simulink model "nonlinear_crane_example"  (Simulink 8.6)
settings: Solver=VariableStepAuto  SolverMode=SingleTasking  StartTime=0.0  StopTime=10  RelTol=1e-3
InitFcn:
  | nonlinear_crane_example_initfcn
values from neighbouring files (symbols this model uses):
  A_nz_idx = ( 1:1:nnz( Anz ) )    [nonlinear_crane_example_initfcn.m]
  Anz = [Anz ... (first row only)    [nonlinear_crane_example_initfcn.m]
  g = 9.81    [nonlinear_crane_example_initfcn.m]
  lineq = repmat(ls, N, 1)    [nonlinear_crane_example_initfcn.m]
  N = 5    [nonlinear_crane_example_initfcn.m]
  nu = 2    [nonlinear_crane_example_initfcn.m]
  nx = 6    [nonlinear_crane_example_initfcn.m]
  P_nz_idx = ( 1:1:nnz( Pnz ) )    [nonlinear_crane_example_initfcn.m]
  Pnz = blkdiag( Pnz, Q )    [nonlinear_crane_example_initfcn.m]
  q = zeros( 1, length(Pnz) )    [nonlinear_crane_example_initfcn.m]
  tau_c = 0.13    [nonlinear_crane_example_initfcn.m]
  tau_l = 0.07    [nonlinear_crane_example_initfcn.m]
  traj_0 = traj_0( 1:1:(length(traj_0)-nu), : )    [nonlinear_crane_example_initfcn.m]
  u0 = zeros(nu, 1)    [nonlinear_crane_example_initfcn.m]
  uineq = repmat(us, N, 1)    [nonlinear_crane_example_initfcn.m]
  x0 = zeros(nx, 1)    [nonlinear_crane_example_initfcn.m]
libraries: osqp_library x1, simulink x1
settings Model: Creator=im1716  LastModifiedBy=imcinerney
settings DataIOCC: LimitDataPoints=off  SaveFormat=Dataset  SignalLoggingSaveFormat=Dataset  ReturnWorkspaceOutputs=on
settings OptimizationCC: ExpressionDepthLimit=128
settings DebuggingCC: UnderspecifiedInitializationDetection=Simplified  MergeDetectMultiDrivingBlocksExec=error  SolverPrmCheckMsg=none  FcnCallInpInsideContextMsg=EnableAllAsError  AllowSymbolicDim=on  StateNameClashWarn=none  SFUnexpectedBacktrackingDiag=error  SFNoUnconditionalDefaultTransitionDiag=error
settings HardwareCC: ProdBitPerPointer=64  ProdLargestAtomicFloat=Float  ProdIntDivRoundTo=Zero  ProdEndianess=LittleEndian  ProdWordSize=64  ProdHWDeviceType=Intel->x86-64 (Windows64)
settings ModelReferenceCC: PropagateSignalLabelsOutOfModel=on
settings SFSimCC: SimUseLocalCustomCode=on
settings RTWCC: RTWUseLocalCustomCode=on
settings GRTTargetCC: TargetLangStandard=C99 (ISO)  GeneratePreprocessorConditionals=Use local settings  CombineOutputUpdateFcns=on  GRTInterface=off
settings ConfigComp: CovMetricSettings=dwe  CovHtmlReporting=off  CovSaveCumulativeToWorkspaceVar=off  CovSaveSingleToWorkspaceVar=off  CovExternalEMLEnable=on

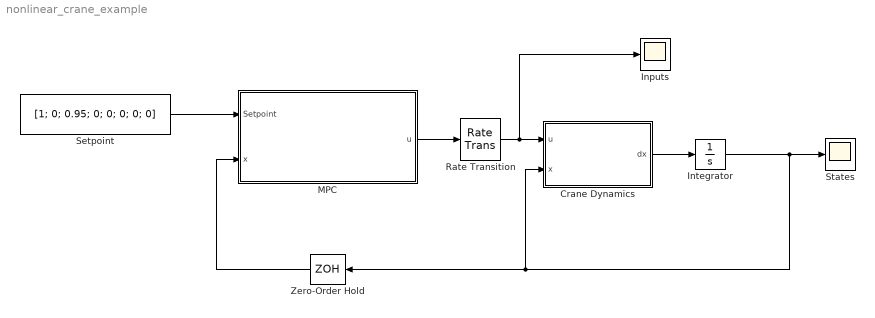
== system nonlinear_crane_example ==
  Crane Dynamics : Subsystem
  Inputs : Scope
  Integrator : Integrator  InitialCondition=x0
  MPC : Subsystem
  Rate Transition : RateTransition  X0=u0
  Setpoint : Constant  Value=[1; 0; 0.95; 0; 0; 0; 0; 0]
  States : Scope
  Zero-Order Hold : ZeroOrderHold  SampleTime=0.001
  wires:
  MPC/1(u) -> Rate Transition/1
  Zero-Order Hold/1 -> MPC/2(x)
  Integrator/1 -> States/1, Crane Dynamics/2(x), Zero-Order Hold/1
  Rate Transition/1 -> Inputs/1, Crane Dynamics/1(u)
  Crane Dynamics/1(dx) -> Integrator/1
  Setpoint/1 -> MPC/1(Setpoint)

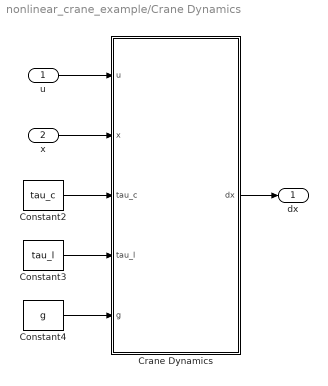
== system nonlinear_crane_example/Crane Dynamics ==
  u : Inport
  x : Inport  Port=2
  Constant2 : Constant  Value=tau_c
  Constant3 : Constant  Value=tau_l
  Constant4 : Constant  Value=g
  Crane Dynamics : MATLAB Function  TreatAsAtomicUnit=on
  dx : Outport
  wires:
  u/1 -> Crane Dynamics/1(u)
  Crane Dynamics/1(dx) -> dx/1
  x/1 -> Crane Dynamics/2(x)
  Constant2/1 -> Crane Dynamics/3(tau_c)
  Constant3/1 -> Crane Dynamics/4(tau_l)
  Constant4/1 -> Crane Dynamics/5(g)

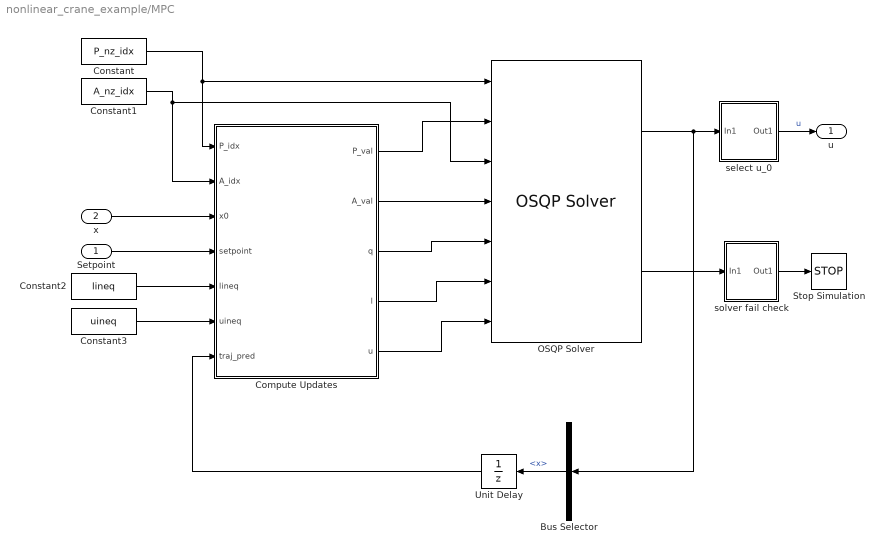
== system nonlinear_crane_example/MPC ==
  Setpoint : Inport
  x : Inport  Port=2
  Bus Selector : BusSelector  OutputSignals=x
  Compute Updates : MATLAB Function  TreatAsAtomicUnit=on
  Constant : Constant  Value=P_nz_idx
  Constant1 : Constant  Value=A_nz_idx
  Constant2 : Constant  Value=lineq
  Constant3 : Constant  Value=uineq
  OSQP Solver : osqp_library/OSQP Solver  P=Pnz  A=Anz  q=q  l=l  u=u  opts={'verbose',true}  refactor_style=Always  warmstart_style=Always  has_external_q_input=on  has_external_bound_input=on  use_custom_osqp_dir=off  dirText=''
  Stop Simulation : Stop
  Unit Delay : UnitDelay  InitialCondition=traj_0  SampleTime=-1  HasFrameUpgradeWarning=on
  select u_0 : Subsystem
  solver fail check : Subsystem
  u : Outport
  wires:
  select u_0/1(Out1) -> u/1  "u"
  solver fail check/1(Out1) -> Stop Simulation/1
  OSQP Solver/2 -> solver fail check/1(In1)
  Compute Updates/5(u) -> OSQP Solver/7
  Compute Updates/4(l) -> OSQP Solver/6
  x/1 -> Compute Updates/3(x0)
  OSQP Solver/1 -> Bus Selector/1, select u_0/1(In1)
  Bus Selector/1 -> Unit Delay/1  "<x>"
  Constant2/1 -> Compute Updates/5(lineq)
  Constant3/1 -> Compute Updates/6(uineq)
  Unit Delay/1 -> Compute Updates/7(traj_pred)
  Constant/1 -> OSQP Solver/1, Compute Updates/1(P_idx)
  Constant1/1 -> Compute Updates/2(A_idx), OSQP Solver/3
  Compute Updates/1(P_val) -> OSQP Solver/2
  Compute Updates/2(A_val) -> OSQP Solver/4
  Setpoint/1 -> Compute Updates/4(setpoint)
  Compute Updates/3(q) -> OSQP Solver/5

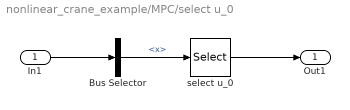
== system nonlinear_crane_example/MPC/select u_0 ==
  In1 : Inport
  Bus Selector : BusSelector  OutputSignals=x
  "select u_0 " : Selector  InputPortWidth=length(q)  IndexOptions=Index vector (dialog)  Indices=((N+1)*nx+1:(N+1)*nx+nu)  OutputSizes=1
  Out1 : Outport
  wires:
  "select u_0 "/1 -> Out1/1
  In1/1 -> Bus Selector/1
  Bus Selector/1 -> "select u_0 "/1  "<x>"

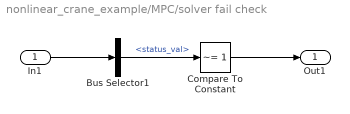
== system nonlinear_crane_example/MPC/solver fail check ==
  In1 : Inport
  Bus Selector1 : BusSelector  OutputSignals=status_val
  Compare To Constant : simulink/Logic and Bit Operations/Compare To Constant  relop=~=  const=1  OutDataTypeStr=boolean
  Out1 : Outport
  wires:
  In1/1 -> Bus Selector1/1
  Compare To Constant/1 -> Out1/1
  Bus Selector1/1 -> Compare To Constant/1  "<status_val>"

== matlab function MPC/Compute Updates ==
  data: P_idx input double; A_idx input double; x0 input double; setpoint input double; lineq input double; uineq input double; P_val output double; A_val output double; q output double; l output double; u output double; traj_pred input double
function [P_val, A_val, q, l, u] = ComputeUpdates( P_idx, A_idx, x0, setpoint, lineq, uineq, traj_pred )

%% Constants for the overhead crane
tau_c = 0.13;
tau_l = 0.07;
g = 9.81;


%% Problem dimensions
N = 5;
nx = 6;
nu = 2;


%% Create the upper/lower bounds
l = [-x0;
      zeros(N*nx, 1);
      lineq];

u = [-x0;
      zeros(N*nx, 1);
      uineq];

h = 0.001;

%% Form the dynamics matrix
A_val = zeros( length(A_idx), 1 );
numA = 16;
numB = 5;
num  = numA + numB;
    
for( i=1:1:N )
    xstart = (nx + nu)*(i-1) + 1;
    xend   = xstart + nx - 1;
    ustart = xend + 1;
    uend   = ustart + nu - 1;
    
    %xp = traj_pred( xstart:1:xend );
    %up = traj_pred( ustart:1:uend );
    xp = traj_pred( 1:1:nx );
    up = traj_pred( nx+1:1:nx+nu+1 );
    
    % Extract the states
    x_c   = xp(1);
    v_c   = xp(2);
    x_l   = xp(3);
    v_l   = xp(4);
    theta = xp(5);
    omega = xp(6);

    % Extract the inputs
    u_c = up(1);
    u_l = up(2);
    
    A = [-1;             % I(1, 1)
          
         -1;             % I(2, 2)
          h*1;             % A(1, 2)
         -h*1 / tau_c;     % A(2, 2)
         -h*cos(theta)/(tau_c*x_l); % A(6, 2)
         
         -1;             % I(3, 3)
         -h*(2*omega*v_l + g*sin(theta) + (cos(theta)*(u_c - v_c))/tau_c)/x_l^2;   % A(6, 3)
          
         -1;             % I(4, 4)
          h*1;             % A(3, 4)
         -h*1 / tau_l;     % A(4, 4)
          h*(2*omega)/x_l; % A(6, 4)
         
         -1;             % I(5, 5)
          h*(g*cos(theta) - (sin(theta)*(u_c - v_c))/tau_c)/x_l;    % A(6, 5)
         
         -1;             % I(6, 6)
          h*1;             % A(5, 6)
          h*2*v_l/x_l];    % A(6, 6)

    B = [ h*1/tau_c; % B(2, 1)
          h*cos(theta)/(tau_c*x_l);  % B(6, 1)
          1;       % E(1, 7)
          
          h*1/tau_l; % B(4, 2)
          1];      % E(2, 8)
    
    istart = num*(i-1)+1;
    iend   = istart + numA-1;
    A_val( istart:1:iend ) = A;

    istart = iend + 1;
    iend   = istart + numB - 1;
    A_val( istart:1:iend ) = B;
end

% The terminal state equality
A = [-1;            % I(1, 1)
     -1;            % I(2, 2)
     -1;            % I(3, 3)
     -1;            % I(4, 4)
     -1;            % I(5, 5)
     -1];           % I(6, 6)
A_val( end-nx+1:1:end ) = A;


%% Just make the P matrix all 1s
Q = diag( [10^(-5), 10^(-5), 10^(-5), 10^(-5), 10^(-5), 10^(-5)] );
R = diag( [10^(-5), 10^(-5)] );
%Q = eye(nx);
%R = eye(nu);

P = kron( eye(N), blkdiag(Q, R) );
P = blkdiag( P, Q );

P_val = diag( P );


%% Create the linear (q) term of the cost
xr = zeros( length(P), 1);
xr(1:end-nx, 1) = repmat( setpoint, N, 1);
xr(end-nx+1:end, 1) = setpoint(1:nx, 1);
q = -2*xr'*P;
%q = zeros( 1, length(q) );

end

== matlab function Crane Dynamics/Crane Dynamics ==
  data: u input double; x input double; dx output double; tau_c input double; tau_l input double; g input double
function dx = craneDynamics( u, x, tau_c, tau_l, g )

% Extract the states
x_c   = x(1);
v_c   = x(2);
x_l   = x(3);
v_l   = x(4);
theta = x(5);
omega = x(6);

% Extract the inputs
u_c = u(1);
u_l = u(2);


%% Compute the derivatives
dot_xc = v_c;
dot_vc = 1/tau_c * (-v_c + u_c);
dot_xl = v_l;
dot_vl = 1/tau_l * (-v_l + u_l);
dot_theta = omega;
dot_omega = 1/x_l * ( (-v_c+u_c)/tau_c*cos(theta) + g*sin(theta) + 2*v_l*omega );


%% Package the derivatives to send out
dx = [dot_xc;
      dot_vc;
      dot_xl;
      dot_vl;
      dot_theta;
      dot_omega];
